simulink model "inv1"  (R2024b)
settings: Solver=VariableStepAuto  StartTime=0.0  StopTime=0.5  MaxStep=1e-6  RelTol=1e-3
libraries: spsMosfetLib x6, spsOnDelayLib x6, spsCurrentMeasurementLib x3, spsDCVoltageSourceLib x3, spsThreePhaseSeriesRLCBranchLib x2, spsVoltageMeasurementLib x2, simulink x1, sps_lib x1
settings Model: Creator=dsz  LastModifiedBy=dsz
settings DataIOCC: ReturnWorkspaceOutputs=off

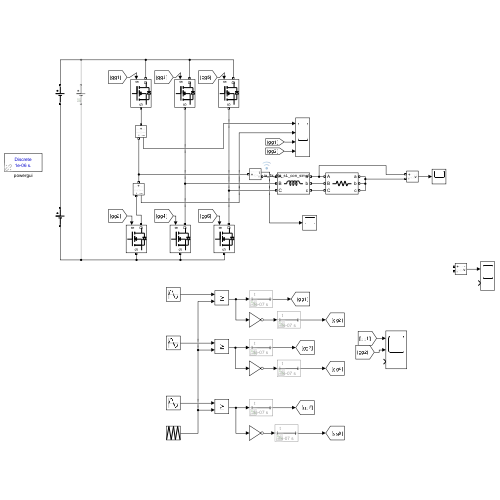
[thumbnail: Simulink's stored preview of the top-level diagram]
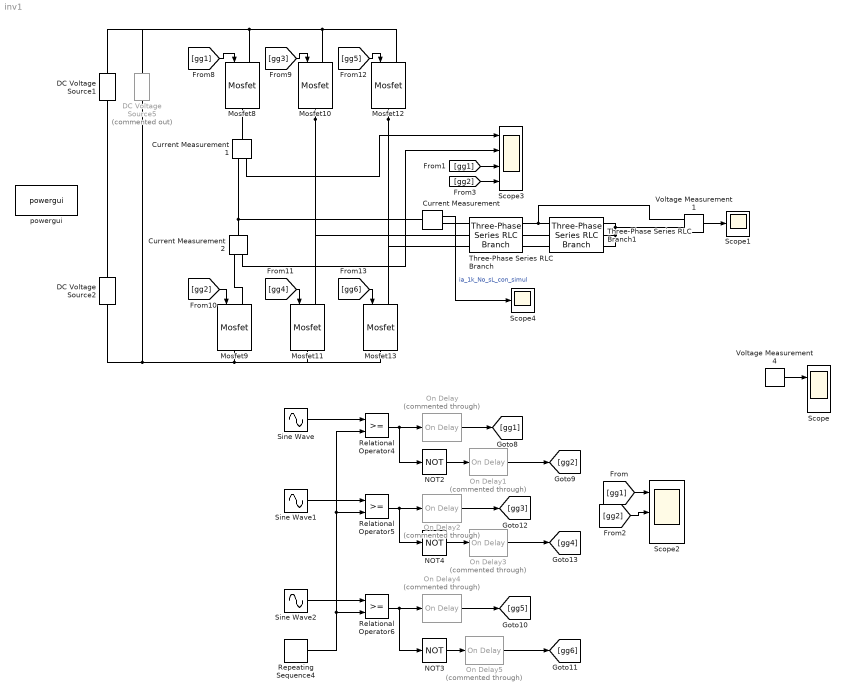
== system inv1 ==
  Current Measurement : spsCurrentMeasurementLib/Current Measurement  PhasorSimulation=off  OutputType=Complex  PSBequivalent=0
  Current Measurement1 : spsCurrentMeasurementLib/Current Measurement  PhasorSimulation=off  OutputType=Complex  PSBequivalent=0
  Current Measurement2 : spsCurrentMeasurementLib/Current Measurement  PhasorSimulation=off  OutputType=Complex  PSBequivalent=0
  DC Voltage Source1 : spsDCVoltageSourceLib/DC Voltage Source  Amplitude=50  Measurements=None
  DC Voltage Source2 : spsDCVoltageSourceLib/DC Voltage Source  Amplitude=50  Measurements=None
  DC Voltage Source5 : spsDCVoltageSourceLib/DC Voltage Source  Commented=on  Amplitude=100  Measurements=None
  Mosfet{8..13} (6 alike) : spsMosfetLib/Mosfet  Ron=0.01  Lon=0  Rd=0.01  Vfd=0  IC=0  Rs=1e5  Cs=inf  Measurements=off
  NOT2 : Logic  Operator=NOT  IconShape=distinctive  AllPortsSameDT=off  OutDataTypeStr=boolean
  NOT3 : Logic  Operator=NOT  IconShape=distinctive  AllPortsSameDT=off  OutDataTypeStr=boolean
  NOT4 : Logic  Operator=NOT  IconShape=distinctive  AllPortsSameDT=off  OutDataTypeStr=boolean
  On Delay{,1..5} (6 alike) : spsOnDelayLib/On Delay  Commented=through  DelayType=On delay  delay=300e-9  ic=0  Ts=0
  Relational Operator4 : RelationalOperator  OutDataTypeStr=boolean  RndMeth=Simplest  InputSameDT=off
  Relational Operator5 : RelationalOperator  OutDataTypeStr=boolean  RndMeth=Simplest  InputSameDT=off
  Relational Operator6 : RelationalOperator  OutDataTypeStr=boolean  RndMeth=Simplest  InputSameDT=off
  Repeating Sequence4 : simulink/Sources/Repeating Sequence  rep_seq_t=[0 5e-4 1e-3]  rep_seq_y=[-0.5 0.5 -0.5]
  Scope : Scope  NumInputPorts=2
  Scope1 : Scope
  Scope2 : Scope  NumInputPorts=3
  Scope3 : Scope  NumInputPorts=4
  Scope4 : Scope
  Sine Wave : Sin  Amplitude=0.5  Frequency=50*2*pi  SampleTime=0
  Sine Wave1 : Sin  Amplitude=0.5  Frequency=50*2*pi  Phase=2/3*pi  SampleTime=0
  Sine Wave2 : Sin  Amplitude=0.5  Frequency=50*2*pi  Phase=4/3*pi  SampleTime=0
  Three-Phase Series RLC Branch : spsThreePhaseSeriesRLCBranchLib/Three-Phase Series RLC Branch  LConnTagsString=A|B|C  RConnTagsString=A|B|C  BranchType=L  Resistance=10  Inductance=0.003  Capacitance=1e-6  Measurements=Branch voltages and currents
  Three-Phase Series RLC Branch1 : spsThreePhaseSeriesRLCBranchLib/Three-Phase Series RLC Branch  LConnTagsString=A|B|C  RConnTagsString=A|B|C  BranchType=R  Resistance=31.7  Inductance=0.1  Capacitance=1e-6  Measurements=Branch voltages
  Voltage Measurement1 : spsVoltageMeasurementLib/Voltage Measurement  PhasorSimulation=off  OutputType=Complex  PSBequivalent=0
  Voltage Measurement4 : spsVoltageMeasurementLib/Voltage Measurement  PhasorSimulation=off  OutputType=Complex  PSBequivalent=0
  powergui : sps_lib/powergui  Priority=1  SimulationMode=Discrete  SampleTime=1e-6  frequency=60  Iterations=50  frequencyindice=0  Pbase=100e6  ErrMax=1e-4  UnitsV=kV  UnitsW=MW  buscounter=0  FunctionMessages=off  echomessages=off  EnableUseOfTLC=off  CurrentSourceSwitches=off  DisableSnubberDevices=off  DisableRonSwitches=off  DisableVfSwitches=off  DisplayEquations=off  AutomaticDiscreteSolvers=off  SolverType=Tustin/Backward Euler (TBE)  Interpol=off  ExternalGateDelay=off  methode=off  Ts=100  x0status=blocks  SPID=on  SwTol=0  HookPort=off  NonlinearTolerance=1e-4  nMaxIteration=100  ContinueOnMaxIteration=off  RestoreLinks=warning  ResistiveCurrentMeasurement=off  Frange=[0:2:500]  Ylog=off  Xlog=on  ShowGrid=off  save=off  variable=ZData  structure=0  ZoomFFT=off  StartTime=0.0  cycles=1  DisplayStyle=1  fundamental=60  FreqAxis=off  MaxFrequency=1000  frequencyindicesteady=1  RmsSteady=1  display=off
  wires:
  Relational Operator4/1 -> NOT2/1, On Delay/1
  NOT2/1 -> On Delay1/1
  Relational Operator6/1 -> NOT3/1, On Delay4/1
  Sine Wave2/1 -> Relational Operator6/1
  Sine Wave1/1 -> Relational Operator5/1
  Voltage Measurement4/1 -> Scope/1
  Sine Wave/1 -> Relational Operator4/1
  NOT3/1 -> On Delay5/1
  NOT4/1 -> On Delay3/1
  Relational Operator5/1 -> NOT4/1, On Delay2/1
  Repeating Sequence4/1 -> Relational Operator5/2, Relational Operator4/2, Relational Operator6/2
  [gg6] -> Mosfet13/1
  [gg1] -> Mosfet8/1
  [gg5] -> Mosfet12/1
  [gg2] -> Mosfet9/1
  [gg4] -> Mosfet11/1
  [gg3] -> Mosfet10/1
  Voltage Measurement1/1 -> Scope1/1
  On Delay/1 -> [gg1]
  On Delay1/1 -> [gg2]
  On Delay2/1 -> [gg3]
  On Delay3/1 -> [gg4]
  On Delay4/1 -> [gg5]
  On Delay5/1 -> [gg6]
  [gg1] -> Scope2/1
  [gg2] -> Scope2/2
  [gg2] -> Scope3/4
  Current Measurement2/1 -> Scope3/2
  Current Measurement1/1 -> Scope3/1
  [gg1] -> Scope3/3
  Current Measurement/1 -> Scope4/1  "ia_1k_No_sL_con_simul"
  connections:
  Three-Phase Series RLC Branch1/LConn1 -- Voltage Measurement1/LConn1 -- Three-Phase Series RLC Branch/RConn1
  Three-Phase Series RLC Branch1/LConn2 -- Three-Phase Series RLC Branch/RConn2
  Three-Phase Series RLC Branch1/LConn3 -- Three-Phase Series RLC Branch/RConn3
  Three-Phase Series RLC Branch1/RConn1 -- Three-Phase Series RLC Branch1/RConn3 -- Three-Phase Series RLC Branch1/RConn2 -- Voltage Measurement1/LConn2
  Mosfet10/RConn1 -- Mosfet11/LConn1 -- Three-Phase Series RLC Branch/LConn2
  Mosfet12/RConn1 -- Mosfet13/LConn1 -- Three-Phase Series RLC Branch/LConn3
  Mosfet10/LConn1 -- DC Voltage Source1/RConn1 -- DC Voltage Source5/RConn1 -- Mosfet8/LConn1 -- Mosfet12/LConn1
  Mosfet9/RConn1 -- DC Voltage Source2/LConn1 -- DC Voltage Source5/LConn1 -- Mosfet13/RConn1 -- Mosfet11/RConn1
  DC Voltage Source2/RConn1 -- DC Voltage Source1/LConn1
  Current Measurement/RConn1 -- Three-Phase Series RLC Branch/LConn1
  Current Measurement2/RConn1 -- Mosfet9/LConn1
  Current Measurement/LConn1 -- Current Measurement1/RConn1 -- Current Measurement2/LConn1
  Mosfet8/RConn1 -- Current Measurement1/LConn1
